simulink model "chap17_01_10_model"  (R2013b)
settings: Solver=ode3  StartTime=0.0  StopTime=10.0  RelTol=1e-3
settings Model: Creator=sunzx.fnst  LastModifiedBy=sunzx.fnst
settings OptimizationCC: InlineParams=on  OptimizeModelRefInitCode=on  LifeSpan=1
settings RTWCC: SystemTargetFile=ert.tlc  GenCodeOnly=on  TemplateMakefile=ert_default_tmf  Description=Embedded Coder  GenerateReport=on  ProcessScript=ert_make_rtw_hook  IncludeHyperlinkInReport=on  LaunchReport=on
settings CodeAppCC: IgnoreCustomStorageClasses=off
settings ERTTargetCC: CodeReplacementLibrary=ANSI_C  GenerateSampleERTMain=on  ERTCustomFileTemplate=example_file_process.tlc

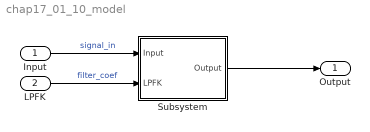
== system chap17_01_10_model ==
  Input : Inport
  LPFK : Inport  Port=2
  Subsystem : Subsystem  TreatAsAtomicUnit=on  RTWFcnName=my_filter  RTWFileName=algorithm_file
      settings: RTWFcnNameOpts=User specified  RTWFileNameOpts=User specified
  Output : Outport
  wires:
  Input/1 -> Subsystem/1(Input)  "signal_in"
  LPFK/1 -> Subsystem/2(LPFK)  "filter_coef"
  Subsystem/1(Output) -> Output/1

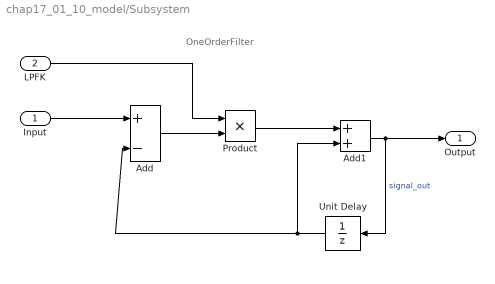
== system chap17_01_10_model/Subsystem ==
  note: OneOrderFilter
  Input : Inport
  LPFK : Inport  Port=2
  Add : Sum  Inputs=+-
  Add1 : Sum
  Product : Product
  Unit Delay : UnitDelay  SampleTime=0.2  StateName=signal_out_old
      settings: CodeGenStateStorageClass=ExportedGlobal
  Output : Outport
  wires:
  Unit Delay/1 -> Add/2, Add1/2
  LPFK/1 -> Product/1
  Product/1 -> Add1/1
  Add/1 -> Product/2
  Input/1 -> Add/1
  Add1/1 -> Unit Delay/1, Output/1  "signal_out"
